simulink model "furuta_model"  (R2025a)
settings: Solver=VariableStepAuto  StartTime=0.0  StopTime=50  RelTol=1e-3
libraries: slpidlib x4
settings Model: Creator=deng_zhiwen  LastModifiedBy=deng_zhiwen

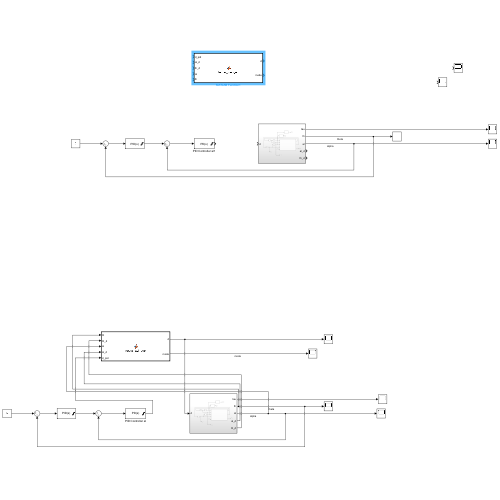
[thumbnail: Simulink's stored preview of the top-level diagram]
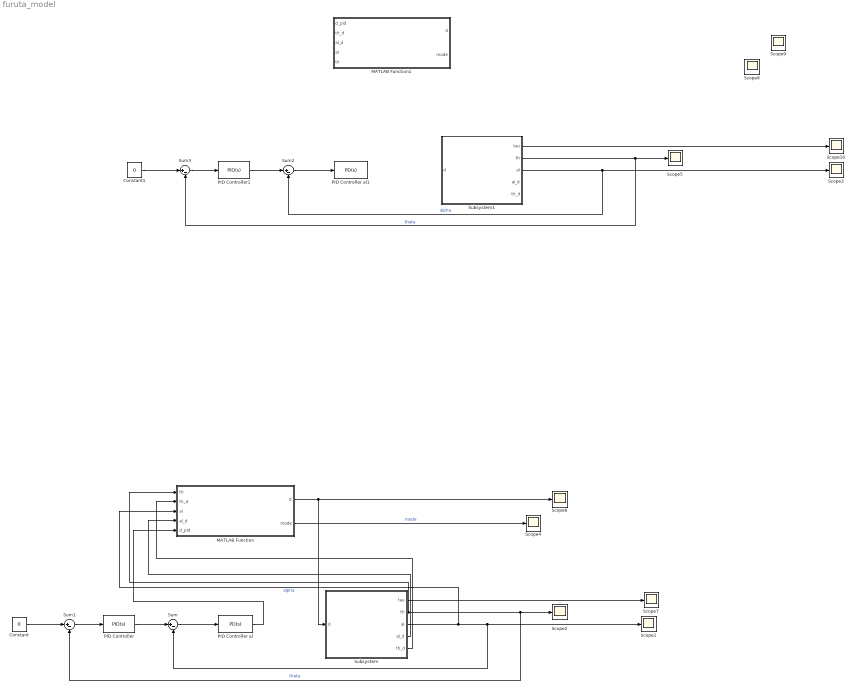
== system furuta_model ==
  Constant : Constant  Value=0
  Constant1 : Constant  Value=0
  MATLAB Function : MATLAB Function  TreatAsAtomicUnit=on
  MATLAB Function1 : MATLAB Function  TreatAsAtomicUnit=on
  PID Controller : slpidlib/PID Controller  Controller=PID  Form=Parallel  TimeDomain=Continuous-time  UseExternalTs=off  SampleTime=-1  IntegratorMethod=Forward Euler  FilterMethod=Forward Euler  ControllerParametersSource=internal  P=0.075  I=0.004  UseKiTs=off  D=0.041  UseExternalDerivativeSource=off  N=100  UseFilter=on  TunerSelectOption=Transfer Function Based (PID Tuner App)  InitialConditionSource=internal  InitialConditionForIntegrator=0  InitialConditionForFilter=0  DifferentiatorICPrevScaledInput=0  ExternalReset=none  TrackingMode=off  Kt=1  LimitOutput=on  SatLimitsSource=internal  UpperSaturationLimit=0.4  LowerSaturationLimit=-0.4  LinearizeAsGain=on  AntiWindupMode=none  Kb=1  LimitIntegrator=off  UpperIntegratorSaturationLimit=inf  LowerIntegratorSaturationLimit=-inf  POutMin=[]  POutMax=[]  IOutMin=[]  IOutMax=[]  DOutMin=[]  DOutMax=[]  NOutMin=[]  NOutMax=[]  SumOutMin=[]  SumOutMax=[]  SaturationOutMin=[]  SaturationOutMax=[]  PParamMin=[]  PParamMax=[]  IParamMin=[]  IParamMax=[]  DParamMin=[]  DParamMax=[]  NParamMin=[]  NParamMax=[]  KbParamMin=[]  KbParamMax=[]  KtParamMin=[]  KtParamMax=[]  KbOutMin=[]  KbOutMax=[]  KtOutMin=[]  KtOutMax=[]  IntegratorOutMin=[]  IntegratorOutMax=[]  FilterOutMin=[]  FilterOutMax=[]  SumI1OutMin=[]  SumI1OutMax=[]  SumI2OutMin=[]  SumI2OutMax=[]  SumI3OutMin=[]  SumI3OutMax=[]  SumI4OutMin=[]  SumI4OutMax=[]  SumDOutMin=[]  SumDOutMax=[]  DifferentiatorOutMin=[]  DifferentiatorOutMax=[]  FilterDiffOutCoefMin=[]  FilterDiffOutCoefMax=[]  ReciprocalOutMin=[]  ReciprocalOutMax=[]  SumDenOutMin=[]  SumDenOutMax=[]  SumNumOutMin=[]  SumNumOutMax=[]  DivideOutMin=[]  DivideOutMax=[]  UdiffTsProdOutMin=[]  UdiffTsProdOutMax=[]  NTsProdOutMin=[]  NTsProdOutMax=[]  UintegralTsProdOutMin=[]  UintegralTsProdOutMax=[]  UngainTsProdOutMin=[]  UngainTsProdOutMax=[]  ClampingZeroOutDataTypeStr=Inherit: Inherit via back propagation  ClampingZeroOutMin=[]  ClampingZeroOutMax=[]  FilterDenConstantOutDataTypeStr=Inherit: Inherit via back propagation  FilterDenConstantOutMin=[]  FilterDenConstantOutMax=[]  PCopyOutDataTypeStr=Inherit: Inherit via back propagation  PCopyOutMin=[]  PCopyOutMax=[]  NCopyOutDataTypeStr=Inherit: Inherit via back propagation  NCopyOutMin=[]  NCopyOutMax=[]  IntegratorContinuousStateAttributes=''  IntegratorStateMustResolveToSignalObject=off  IntegratorRTWStateStorageClass=Auto  FilterContinuousStateAttributes=''  FilterStateMustResolveToSignalObject=off  FilterRTWStateStorageClass=Auto  ParallelPVariant=InternalParameters  IdealPVariant=Disabled  IVariant=InternalParameters  DVariant=InternalParameters  IntegratorVariant=Continuous  SatVariant=Enabled  AWVariant=Passthrough  PCopyVariant=Disabled  TRVariant=Disabled  FdbkBlocksVariant=Forward  IdealPFdbkVariant=Disabled  SatFdbkVariant=Disabled  DerivativeFilterVariant=ContFilter  NVariant=InternalParameters  NCopyVariant=Disabled  FilterICVariant=InternalICsFilter  IntegratorICVariant=InternalICs  ExternalResetVariant=Disabled  TRSumVariant=Passthrough  SumFdbkVariant=Disabled  SumVariant=Sum_PID  TsampFilterVariant=InternalTs  TsampNgainVariant=Passthrough  TsampIntegralVariant=Disabled_SignalSpec  ExternalSaturationOutDataTypeStr=Inherit: Same as second input  DerivativeSourceVariant=ErrorSignal  PreIntVariant=InternalPreInt
  PID Controller al : slpidlib/PID Controller  Controller=PD  Form=Parallel  TimeDomain=Continuous-time  UseExternalTs=off  SampleTime=-1  IntegratorMethod=Forward Euler  FilterMethod=Forward Euler  ControllerParametersSource=internal  P=-1.37821105216692  I=-0.127510528430422  UseKiTs=off  D=-0.100817816501645  UseExternalDerivativeSource=off  N=47.2284869884382  UseFilter=on  TunerSelectOption=Transfer Function Based (PID Tuner App)  InitialConditionSource=internal  InitialConditionForIntegrator=0  InitialConditionForFilter=0  DifferentiatorICPrevScaledInput=0  ExternalReset=none  TrackingMode=off  Kt=1  LimitOutput=on  SatLimitsSource=internal  UpperSaturationLimit=1  LowerSaturationLimit=-1  LinearizeAsGain=on  AntiWindupMode=none  Kb=1  LimitIntegrator=off  UpperIntegratorSaturationLimit=inf  LowerIntegratorSaturationLimit=-inf  POutMin=[]  POutMax=[]  IOutMin=[]  IOutMax=[]  DOutMin=[]  DOutMax=[]  NOutMin=[]  NOutMax=[]  SumOutMin=[]  SumOutMax=[]  SaturationOutMin=[]  SaturationOutMax=[]  PParamMin=[]  PParamMax=[]  IParamMin=[]  IParamMax=[]  DParamMin=[]  DParamMax=[]  NParamMin=[]  NParamMax=[]  KbParamMin=[]  KbParamMax=[]  KtParamMin=[]  KtParamMax=[]  KbOutMin=[]  KbOutMax=[]  KtOutMin=[]  KtOutMax=[]  IntegratorOutMin=[]  IntegratorOutMax=[]  FilterOutMin=[]  FilterOutMax=[]  SumI1OutMin=[]  SumI1OutMax=[]  SumI2OutMin=[]  SumI2OutMax=[]  SumI3OutMin=[]  SumI3OutMax=[]  SumI4OutMin=[]  SumI4OutMax=[]  SumDOutMin=[]  SumDOutMax=[]  DifferentiatorOutMin=[]  DifferentiatorOutMax=[]  FilterDiffOutCoefMin=[]  FilterDiffOutCoefMax=[]  ReciprocalOutMin=[]  ReciprocalOutMax=[]  SumDenOutMin=[]  SumDenOutMax=[]  SumNumOutMin=[]  SumNumOutMax=[]  DivideOutMin=[]  DivideOutMax=[]  UdiffTsProdOutMin=[]  UdiffTsProdOutMax=[]  NTsProdOutMin=[]  NTsProdOutMax=[]  UintegralTsProdOutMin=[]  UintegralTsProdOutMax=[]  UngainTsProdOutMin=[]  UngainTsProdOutMax=[]  ClampingZeroOutDataTypeStr=Inherit: Inherit via back propagation  ClampingZeroOutMin=[]  ClampingZeroOutMax=[]  FilterDenConstantOutDataTypeStr=Inherit: Inherit via back propagation  FilterDenConstantOutMin=[]  FilterDenConstantOutMax=[]  PCopyOutDataTypeStr=Inherit: Inherit via back propagation  PCopyOutMin=[]  PCopyOutMax=[]  NCopyOutDataTypeStr=Inherit: Inherit via back propagation  NCopyOutMin=[]  NCopyOutMax=[]  IntegratorContinuousStateAttributes=''  IntegratorStateMustResolveToSignalObject=off  IntegratorRTWStateStorageClass=Auto  FilterContinuousStateAttributes=''  FilterStateMustResolveToSignalObject=off  FilterRTWStateStorageClass=Auto  ParallelPVariant=InternalParameters  IdealPVariant=Disabled  IVariant=Disabled  DVariant=InternalParameters  IntegratorVariant=Disabled  SatVariant=Enabled  AWVariant=Disabled  PCopyVariant=Disabled  TRVariant=Disabled  FdbkBlocksVariant=Forward  IdealPFdbkVariant=Disabled  SatFdbkVariant=Disabled  DerivativeFilterVariant=ContFilter  NVariant=InternalParameters  NCopyVariant=Disabled  FilterICVariant=InternalICsFilter  IntegratorICVariant=Disabled  ExternalResetVariant=Disabled  TRSumVariant=Passthrough  SumFdbkVariant=Disabled  SumVariant=Sum_PD  TsampFilterVariant=InternalTs  TsampNgainVariant=Passthrough  TsampIntegralVariant=Disabled_SignalSpec  ExternalSaturationOutDataTypeStr=Inherit: Same as second input  DerivativeSourceVariant=ErrorSignal  PreIntVariant=InternalPreInt
  PID Controller al1 : slpidlib/PID Controller  Controller=PD  Form=Parallel  TimeDomain=Continuous-time  UseExternalTs=off  SampleTime=-1  IntegratorMethod=Forward Euler  FilterMethod=Forward Euler  ControllerParametersSource=internal  P=-1.37821105216692  I=-0.127510528430422  UseKiTs=off  D=-0.100817816501645  UseExternalDerivativeSource=off  N=47.2284869884382  UseFilter=on  TunerSelectOption=Transfer Function Based (PID Tuner App)  InitialConditionSource=internal  InitialConditionForIntegrator=0  InitialConditionForFilter=0  DifferentiatorICPrevScaledInput=0  ExternalReset=none  TrackingMode=off  Kt=1  LimitOutput=on  SatLimitsSource=internal  UpperSaturationLimit=1  LowerSaturationLimit=-1  LinearizeAsGain=on  AntiWindupMode=none  Kb=1  LimitIntegrator=off  UpperIntegratorSaturationLimit=inf  LowerIntegratorSaturationLimit=-inf  POutMin=[]  POutMax=[]  IOutMin=[]  IOutMax=[]  DOutMin=[]  DOutMax=[]  NOutMin=[]  NOutMax=[]  SumOutMin=[]  SumOutMax=[]  SaturationOutMin=[]  SaturationOutMax=[]  PParamMin=[]  PParamMax=[]  IParamMin=[]  IParamMax=[]  DParamMin=[]  DParamMax=[]  NParamMin=[]  NParamMax=[]  KbParamMin=[]  KbParamMax=[]  KtParamMin=[]  KtParamMax=[]  KbOutMin=[]  KbOutMax=[]  KtOutMin=[]  KtOutMax=[]  IntegratorOutMin=[]  IntegratorOutMax=[]  FilterOutMin=[]  FilterOutMax=[]  SumI1OutMin=[]  SumI1OutMax=[]  SumI2OutMin=[]  SumI2OutMax=[]  SumI3OutMin=[]  SumI3OutMax=[]  SumI4OutMin=[]  SumI4OutMax=[]  SumDOutMin=[]  SumDOutMax=[]  DifferentiatorOutMin=[]  DifferentiatorOutMax=[]  FilterDiffOutCoefMin=[]  FilterDiffOutCoefMax=[]  ReciprocalOutMin=[]  ReciprocalOutMax=[]  SumDenOutMin=[]  SumDenOutMax=[]  SumNumOutMin=[]  SumNumOutMax=[]  DivideOutMin=[]  DivideOutMax=[]  UdiffTsProdOutMin=[]  UdiffTsProdOutMax=[]  NTsProdOutMin=[]  NTsProdOutMax=[]  UintegralTsProdOutMin=[]  UintegralTsProdOutMax=[]  UngainTsProdOutMin=[]  UngainTsProdOutMax=[]  ClampingZeroOutDataTypeStr=Inherit: Inherit via back propagation  ClampingZeroOutMin=[]  ClampingZeroOutMax=[]  FilterDenConstantOutDataTypeStr=Inherit: Inherit via back propagation  FilterDenConstantOutMin=[]  FilterDenConstantOutMax=[]  PCopyOutDataTypeStr=Inherit: Inherit via back propagation  PCopyOutMin=[]  PCopyOutMax=[]  NCopyOutDataTypeStr=Inherit: Inherit via back propagation  NCopyOutMin=[]  NCopyOutMax=[]  IntegratorContinuousStateAttributes=''  IntegratorStateMustResolveToSignalObject=off  IntegratorRTWStateStorageClass=Auto  FilterContinuousStateAttributes=''  FilterStateMustResolveToSignalObject=off  FilterRTWStateStorageClass=Auto  ParallelPVariant=InternalParameters  IdealPVariant=Disabled  IVariant=Disabled  DVariant=InternalParameters  IntegratorVariant=Disabled  SatVariant=Enabled  AWVariant=Disabled  PCopyVariant=Disabled  TRVariant=Disabled  FdbkBlocksVariant=Forward  IdealPFdbkVariant=Disabled  SatFdbkVariant=Disabled  DerivativeFilterVariant=ContFilter  NVariant=InternalParameters  NCopyVariant=Disabled  FilterICVariant=InternalICsFilter  IntegratorICVariant=Disabled  ExternalResetVariant=Disabled  TRSumVariant=Passthrough  SumFdbkVariant=Disabled  SumVariant=Sum_PD  TsampFilterVariant=InternalTs  TsampNgainVariant=Passthrough  TsampIntegralVariant=Disabled_SignalSpec  ExternalSaturationOutDataTypeStr=Inherit: Same as second input  DerivativeSourceVariant=ErrorSignal  PreIntVariant=InternalPreInt
  PID Controller1 : slpidlib/PID Controller  Controller=PID  Form=Parallel  TimeDomain=Continuous-time  UseExternalTs=off  SampleTime=-1  IntegratorMethod=Forward Euler  FilterMethod=Forward Euler  ControllerParametersSource=internal  P=0.075  I=0.004  UseKiTs=off  D=0.041  UseExternalDerivativeSource=off  N=100  UseFilter=on  TunerSelectOption=Transfer Function Based (PID Tuner App)  InitialConditionSource=internal  InitialConditionForIntegrator=0  InitialConditionForFilter=0  DifferentiatorICPrevScaledInput=0  ExternalReset=none  TrackingMode=off  Kt=1  LimitOutput=on  SatLimitsSource=internal  UpperSaturationLimit=0.4  LowerSaturationLimit=-0.4  LinearizeAsGain=on  AntiWindupMode=none  Kb=1  LimitIntegrator=off  UpperIntegratorSaturationLimit=inf  LowerIntegratorSaturationLimit=-inf  POutMin=[]  POutMax=[]  IOutMin=[]  IOutMax=[]  DOutMin=[]  DOutMax=[]  NOutMin=[]  NOutMax=[]  SumOutMin=[]  SumOutMax=[]  SaturationOutMin=[]  SaturationOutMax=[]  PParamMin=[]  PParamMax=[]  IParamMin=[]  IParamMax=[]  DParamMin=[]  DParamMax=[]  NParamMin=[]  NParamMax=[]  KbParamMin=[]  KbParamMax=[]  KtParamMin=[]  KtParamMax=[]  KbOutMin=[]  KbOutMax=[]  KtOutMin=[]  KtOutMax=[]  IntegratorOutMin=[]  IntegratorOutMax=[]  FilterOutMin=[]  FilterOutMax=[]  SumI1OutMin=[]  SumI1OutMax=[]  SumI2OutMin=[]  SumI2OutMax=[]  SumI3OutMin=[]  SumI3OutMax=[]  SumI4OutMin=[]  SumI4OutMax=[]  SumDOutMin=[]  SumDOutMax=[]  DifferentiatorOutMin=[]  DifferentiatorOutMax=[]  FilterDiffOutCoefMin=[]  FilterDiffOutCoefMax=[]  ReciprocalOutMin=[]  ReciprocalOutMax=[]  SumDenOutMin=[]  SumDenOutMax=[]  SumNumOutMin=[]  SumNumOutMax=[]  DivideOutMin=[]  DivideOutMax=[]  UdiffTsProdOutMin=[]  UdiffTsProdOutMax=[]  NTsProdOutMin=[]  NTsProdOutMax=[]  UintegralTsProdOutMin=[]  UintegralTsProdOutMax=[]  UngainTsProdOutMin=[]  UngainTsProdOutMax=[]  ClampingZeroOutDataTypeStr=Inherit: Inherit via back propagation  ClampingZeroOutMin=[]  ClampingZeroOutMax=[]  FilterDenConstantOutDataTypeStr=Inherit: Inherit via back propagation  FilterDenConstantOutMin=[]  FilterDenConstantOutMax=[]  PCopyOutDataTypeStr=Inherit: Inherit via back propagation  PCopyOutMin=[]  PCopyOutMax=[]  NCopyOutDataTypeStr=Inherit: Inherit via back propagation  NCopyOutMin=[]  NCopyOutMax=[]  IntegratorContinuousStateAttributes=''  IntegratorStateMustResolveToSignalObject=off  IntegratorRTWStateStorageClass=Auto  FilterContinuousStateAttributes=''  FilterStateMustResolveToSignalObject=off  FilterRTWStateStorageClass=Auto  ParallelPVariant=InternalParameters  IdealPVariant=Disabled  IVariant=InternalParameters  DVariant=InternalParameters  IntegratorVariant=Continuous  SatVariant=Enabled  AWVariant=Passthrough  PCopyVariant=Disabled  TRVariant=Disabled  FdbkBlocksVariant=Forward  IdealPFdbkVariant=Disabled  SatFdbkVariant=Disabled  DerivativeFilterVariant=ContFilter  NVariant=InternalParameters  NCopyVariant=Disabled  FilterICVariant=InternalICsFilter  IntegratorICVariant=InternalICs  ExternalResetVariant=Disabled  TRSumVariant=Passthrough  SumFdbkVariant=Disabled  SumVariant=Sum_PID  TsampFilterVariant=InternalTs  TsampNgainVariant=Passthrough  TsampIntegralVariant=Disabled_SignalSpec  ExternalSaturationOutDataTypeStr=Inherit: Same as second input  DerivativeSourceVariant=ErrorSignal  PreIntVariant=InternalPreInt
  Scope{1..10} (10 alike) : Scope
      Scope1 settings: ActiveDisplayYMinimum=-3.9269908169872414  ActiveDisplayYMaximum=3.9269908169872414
      Scope10 settings: ActiveDisplayYMinimum=-1  ActiveDisplayYMaximum=1  DataLoggingVariableName=ScopeData3
      Scope2 settings: ActiveDisplayYMinimum=-3.9269908169872245  ActiveDisplayYMaximum=3.926990816987229  DataLoggingVariableName=ScopeData2
      Scope3 settings: ActiveDisplayYMinimum=-3.9269908169872414  ActiveDisplayYMaximum=3.9269908169872414  DataLoggingVariableName=ScopeData4
      Scope4 settings: ActiveDisplayYMinimum=-0.15834947271429556  ActiveDisplayYMaximum=1.034336584628718
      Scope5 settings: ActiveDisplayYMinimum=-3.9269908169872245  ActiveDisplayYMaximum=3.926990816987229  DataLoggingVariableName=ScopeData5
      Scope6 settings: ActiveDisplayYMinimum=-1.4910481407596079  ActiveDisplayYMaximum=1.3792930645972798  DataLoggingVariableName=ScopeData6
      Scope7 settings: ActiveDisplayYMinimum=-1  ActiveDisplayYMaximum=1  DataLoggingVariableName=ScopeData7
      Scope8 settings: ActiveDisplayYMinimum=-0.15834947271429556  ActiveDisplayYMaximum=1.034336584628718  DataLoggingVariableName=ScopeData8
      Scope9 settings: ActiveDisplayYMinimum=-1.4910481407596079  ActiveDisplayYMaximum=1.3792930645972798  DataLoggingVariableName=ScopeData9
  Subsystem : Subsystem
  Subsystem1 : Subsystem
  Sum{,1..3} (4 alike) : Sum  Inputs=|+-
  wires:
  Subsystem/2(th) -> MATLAB Function/1(th), Sum1/2, Scope2/1  "theta"
  Constant/1 -> Sum1/1
  PID Controller/1 -> Sum/1
  Sum1/1 -> PID Controller/1
  Sum/1 -> PID Controller al/1
  Subsystem/3(al) -> Sum/2, Scope1/1, MATLAB Function/3(al)  "alpha"
  Subsystem/5(th_d) -> MATLAB Function/2(th_d)
  Subsystem/4(al_d) -> MATLAB Function/4(al_d)
  MATLAB Function/1(d) -> Scope6/1, Subsystem/1(d)
  PID Controller al/1 -> MATLAB Function/5(d_pid)
  MATLAB Function/2(mode) -> Scope4/1  "mode"
  Subsystem/1(tau) -> Scope7/1
  Subsystem1/2(th) -> Sum3/2, Scope5/1  "theta"
  PID Controller1/1 -> Sum2/1
  Subsystem1/1(tau) -> Scope10/1
  Constant1/1 -> Sum3/1
  Sum3/1 -> PID Controller1/1
  Subsystem1/3(al) -> Sum2/2, Scope3/1  "alpha"
  Sum2/1 -> PID Controller al1/1

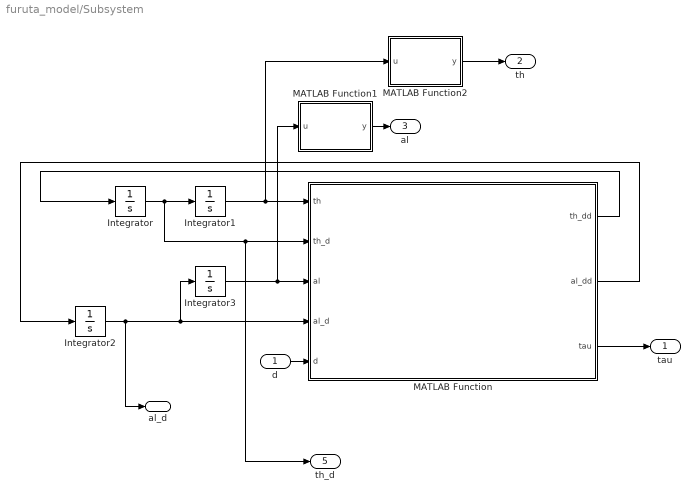
== system furuta_model/Subsystem ==
  d : Inport
  Integrator : Integrator
  Integrator1 : Integrator
  Integrator2 : Integrator  InitialCondition=0.3
  Integrator3 : Integrator  InitialCondition=0.24
  MATLAB Function : MATLAB Function  TreatAsAtomicUnit=on
  MATLAB Function1 : MATLAB Function  TreatAsAtomicUnit=on
  MATLAB Function2 : MATLAB Function  TreatAsAtomicUnit=on
  tau : Outport
  th : Outport  Port=2
  al : Outport  Port=3
  al_d : Outport  Port=4
  th_d : Outport  Port=5
  wires:
  MATLAB Function/1(th_dd) -> Integrator/1
  MATLAB Function/2(al_dd) -> Integrator2/1
  Integrator/1 -> Integrator1/1, MATLAB Function/2(th_d), th_d/1
  d/1 -> MATLAB Function/5(d)
  Integrator2/1 -> MATLAB Function/4(al_d), Integrator3/1, al_d/1
  MATLAB Function/3(tau) -> tau/1
  Integrator1/1 -> MATLAB Function2/1(u), MATLAB Function/1(th)
  Integrator3/1 -> MATLAB Function1/1(u), MATLAB Function/3(al)
  MATLAB Function1/1(y) -> al/1
  MATLAB Function2/1(y) -> th/1

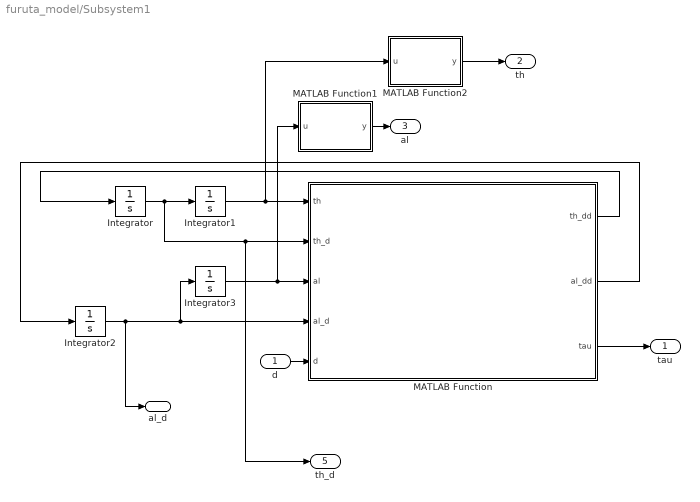
== system furuta_model/Subsystem1 ==
  d : Inport
  Integrator : Integrator
  Integrator1 : Integrator
  Integrator2 : Integrator  InitialCondition=0.3
  Integrator3 : Integrator  InitialCondition=0.24
  MATLAB Function : MATLAB Function  TreatAsAtomicUnit=on
  MATLAB Function1 : MATLAB Function  TreatAsAtomicUnit=on
  MATLAB Function2 : MATLAB Function  TreatAsAtomicUnit=on
  tau : Outport
  th : Outport  Port=2
  al : Outport  Port=3
  al_d : Outport  Port=4
  th_d : Outport  Port=5
  wires:
  MATLAB Function/1(th_dd) -> Integrator/1
  MATLAB Function/2(al_dd) -> Integrator2/1
  Integrator/1 -> Integrator1/1, MATLAB Function/2(th_d), th_d/1
  d/1 -> MATLAB Function/5(d)
  Integrator2/1 -> MATLAB Function/4(al_d), Integrator3/1, al_d/1
  MATLAB Function/3(tau) -> tau/1
  Integrator1/1 -> MATLAB Function2/1(u), MATLAB Function/1(th)
  Integrator3/1 -> MATLAB Function1/1(u), MATLAB Function/3(al)
  MATLAB Function1/1(y) -> al/1
  MATLAB Function2/1(y) -> th/1

== matlab function furuta_model/Subsystem/MATLAB Function1 ==
  data: u input; y output
function y = wrap_angle(u)
    y = atan2(sin(u), cos(u));
end

== matlab function furuta_model/Subsystem/MATLAB Function ==
  data: th input; th_dd output; th_d input; al input; al_d input; d input; al_dd output; tau output
function [th_dd, al_dd, tau] = furuta_step(th, th_d, al, al_d, d)
%#codegen
% States: th=theta, th_d=theta_dot, al=alpha, al_d=alpha_dot
% Input:  d = PWM duty [-1, 1]
% Output: th_dd, al_dd [rad/s²], tau [N·m]

% -------------------------------------------------------------------------
% 物理参数
% -------------------------------------------------------------------------
J_theta = 2.5e-4;   % 旋转臂转动惯量        [kg·m²]
J_alpha = 1.2e-3;   % 摆杆转动惯量          [kg·m²]
m_p     = 0.120;    % 摆杆质量              [kg]
r       = 0.1;      % 旋转臂长度            [m]
l       = 0.1;      % 摆杆质心到摆轴距离    [m]
g       = 9.81;     % 重力加速度            [m/s²]
B_r     = 0.0024;   % 旋转臂阻尼系数        [N·m·s/rad]
B_p     = 0.0024;   % 摆轴阻尼系数          [N·m·s/rad]

% 电机参数
K_g     = 9.2767;   % 减速比
V_s     = 5.0;      % 供电电压              [V]
R_m     = 2.5;      % 电枢电阻              [Ω]
k_t     = 0.020;    % 力矩常数              [N·m/A]
k_e     = 0.020;    % 反电动势常数          [V·s/rad]
eta_m   = 0.7;      % 电机效率
eta_g   = 0.7;      % 减速箱效率
tau_max = 0.25;     % 力矩饱和值            [N·m]

% -------------------------------------------------------------------------
% 动力学方程组合参数（从物理参数推导，便于核查）
%
%   惯性矩阵 M = [a,        e*cos(al)]
%               [e*cos(al), c        ]
%
%   a  = J_theta + m_p*r²   旋转臂等效惯量
%   c  = J_alpha + m_p*l²   摆杆等效惯量
%   e  = m_p*r*l            耦合项幅值，实际耦合项 b = e*cos(al)
%   g0 = m_p*g*l            重力项幅值，实际重力项 = g0*sin(al)
% -------------------------------------------------------------------------
a  = J_theta + m_p * r^2;   % = 2.5e-4 + 0.12×0.1² = 1.45e-3  [kg·m²]
c  = J_alpha + m_p * l^2;   % = 1.2e-3 + 0.12×0.1² = 2.40e-3  [kg·m²]
e  = m_p * r * l;           % = 0.12×0.1×0.1        = 1.20e-3  [kg·m²]
g0 = m_p * g * l;           % = 0.12×9.81×0.1       = 0.11772  [N·m]

% -------------------------------------------------------------------------
% 力矩计算: tau = eta_m*eta_g*K_g*k_t*(V_s*d - k_e*K_g*th_d) / R_m
%               = Cd*d - Cv*th_d
% -------------------------------------------------------------------------
Cd = eta_m * eta_g * K_g * k_t * V_s / R_m;       % ≈ 0.18182 [N·m/duty]
Cv = eta_m * eta_g * K_g^2 * k_t * k_e / R_m;     % ≈ 0.00675 [N·m·s/rad]

tau_raw = Cd*d - Cv*th_d;
tau     = max(-tau_max, min(tau_max, tau_raw));     % 力矩饱和
% -------------------------------------------------------------------------
% 构建右端向量
%
%   rhs1 = tau - B_r*th_d + e*sin(al)*al_d²    (θ方程，含离心项)
%   rhs2 =     - B_p*al_d + g0*sin(al)          (α方程，含重力项)
% -------------------------------------------------------------------------
b    = e * cos(al);                        % 惯性矩阵耦合项    [kg·m²]

rhs1 = tau - B_r*th_d + e*sin(al)*al_d^2;
rhs2 =     - B_p*al_d + g0*sin(al);

% -------------------------------------------------------------------------
% 克莱姆法则求解 M*[th_dd; al_dd] = [rhs1; rhs2]
%
%   detM = a*c - b²  (恒 > 0，已验证最小值 a*c-e² = 2.04e-6 > 0)
% -------------------------------------------------------------------------
detM  = a*c - b^2;

th_dd = ( c*rhs1 - b*rhs2) / detM;
al_dd = (-b*rhs1 + a*rhs2) / detM;

end

== matlab function furuta_model/Subsystem/MATLAB Function2 ==
  data: u input; y output
function y = wrap_angle(u)
    y = atan2(sin(u), cos(u));
end

== matlab function furuta_model/MATLAB Function ==
  data: th input; d output; th_d input; al input; al_d input; d_pid input; mode output
function [d, mode] = furuta_swingup(th, th_d, al, al_d, d_pid)
%#codegen
% Inputs:
%   th, th_d : 旋转臂角度和角速度 [rad, rad/s]
%   al, al_d : 摆杆角度和角速度 [rad, rad/s] (al=0为倒立，al=+-pi为自然下垂)
%   d_pid    : PID控制器计算出的占空比 (用于在起摆完成后接管)
% Outputs:
%   d        : 最终输出给电机的占空比 [-1, 1]
%   mode     : 当前控制模式 (0: 起摆模式, 1: PID稳态控制模式)

% --- 关键修复：显式初始化输出变量的维度和类型，防止Simulink报错 ---
d = 0.0;
mode = 0;

% -------------------------------------------------------------------------
% 物理参数 (与你的动力学模型完全一致)
% -------------------------------------------------------------------------
J_theta = 2.5e-4;   
J_alpha = 1.2e-3;   
m_p     = 0.120;    
r       = 0.1;      
l       = 0.1;      
g       = 9.81;     
B_r     = 0.0024;   
B_p     = 0.0024;   

% 电机参数
K_g     = 9.2767;   
V_s     = 5.0;      
R_m     = 2.5;      
k_t     = 0.020;    
k_e     = 0.020;    
eta_m   = 0.7;      
eta_g   = 0.7;      

% 动力学组合参数
a  = J_theta + m_p * r^2;
c  = J_alpha + m_p * l^2;
e  = m_p * r * l;
g0 = m_p * g * l;

% 电机模型组合参数
Cd = eta_m * eta_g * K_g * k_t * V_s / R_m;
Cv = eta_m * eta_g * K_g^2 * k_t * k_e / R_m;

% -------------------------------------------------------------------------
% 1. 角度规范化到 [-pi, pi]
% -------------------------------------------------------------------------
% 防止由于多圈旋转导致的角度累加，将 al 限制在 [-pi, pi]
al_wrap = mod(al + pi, 2*pi) - pi;

% -------------------------------------------------------------------------
% 2. 切换逻辑：判断是否进入PID接管范围 (20度)
% -------------------------------------------------------------------------
threshold = 20 * pi / 180; % 20度转化为弧度

if abs(al_wrap) <= threshold
    % --- PID 接管模式 ---
    mode = 1; 
    d = d_pid;
else
    % --- 能量起摆模式 ---
    mode = 0; 
    
    % ---------------------------------------------------------------------
    % 3. 满血版 Bang-Bang 能量控制律 (解决高处回落问题)
    % ---------------------------------------------------------------------
    E = 0.5 * c * al_d^2 + g0 * cos(al);
    
    % 【关键修改1】将目标能量提高到理论最大势能的 1.5 倍！
    % 防止在接近最高点时，控制器认为“能量够了”而提前关断电机，导致被摩擦力消耗掉而掉下来。
    E0 = g0 * 1.5; 
    
    k_acc = 120.0; 
    
    % 【关键修改2】限制旋臂回中力矩的最大值
    % 防止旋臂偏离过大时，PD控制力矩增长过大，喧宾夺主抵消了起摆力矩
    pd_term = 2.0 * th + 2.0 * th_d;
    pd_term = max(-50, min(50, pd_term)); % 强行限幅
    
    pump_direction = sign(al_d * cos(al));
    if pump_direction == 0
        pump_direction = 1; 
    end
    
    % 只要能量不够，就全功率泵入 (由于 E0 设得很高，起摆阶段会一直全功率泵入)
    if E < E0
        th_dd_cmd = -k_acc * pump_direction - pd_term;
    else
        th_dd_cmd = -pd_term; 
    end
    
    % 限制期望加速度
    th_dd_cmd = max(-150, min(150, th_dd_cmd));

    
    % ---------------------------------------------------------------------
    % 4. 逆动力学补偿计算目标力矩 (tau_cmd)
    % ---------------------------------------------------------------------
    b = e * cos(al);
    
    % 根据期望的 th_dd_cmd 预测此时摆杆的角加速度 al_dd
    % 由动力学方程2变形得到: c * al_dd = -b * th_dd - B_p * al_d + g0 * sin(al)
    al_dd_pred = (-b * th_dd_cmd - B_p * al_d + g0 * sin(al)) / c;
    
    % 代入动力学方程1求所需的目标力矩 tau_cmd
    % a * th_dd + b * al_dd = tau - B_r * th_d + e * sin(al) * al_d^2
    tau_cmd = a * th_dd_cmd + b * al_dd_pred + B_r * th_d - e * sin(al) * al_d^2;
    
    % ---------------------------------------------------------------------
    % 5. 逆电机模型补偿计算占空比 (d)
    % ---------------------------------------------------------------------
    % 正向电机模型: tau = Cd * d - Cv * th_d
    % 逆向电机模型: d = (tau + Cv * th_d) / Cd
    d_raw = (tau_cmd + Cv * th_d) / Cd;
    
    % 占空比饱和限制 [-1, 1]
    d = max(-1, min(1, d_raw));
end

end

== matlab function furuta_model/MATLAB Function1 ==
  data: d_pid input; th_d input; al_d input; al input; th input; d output; mode output
function [d, mode] = furuta_swingup(d_pid,th_d,al_d,al,th)
%#codegen
% Inputs:
%   th, th_d : 旋转臂角度和角速度 [rad, rad/s]
%   al, al_d : 摆杆角度和角速度 [rad, rad/s] (al=0为倒立，al=+-pi为自然下垂)
%   d_pid    : PID控制器计算出的占空比 (用于在起摆完成后接管)
% Outputs:
%   d        : 最终输出给电机的占空比 [-1, 1]
%   mode     : 当前控制模式 (0: 起摆模式, 1: PID稳态控制模式)

% --- 关键修复：显式初始化输出变量的维度和类型，防止Simulink报错 ---
d = 0.0;
mode = 0;

% -------------------------------------------------------------------------
% 物理参数 (与你的动力学模型完全一致)
% -------------------------------------------------------------------------
J_theta = 2.5e-4;   
J_alpha = 1.2e-3;   
m_p     = 0.120;    
r       = 0.1;      
l       = 0.1;      
g       = 9.81;     
B_r     = 0.0024;   
B_p     = 0.0024;   

% 电机参数
K_g     = 9.2767;   
V_s     = 5.0;      
R_m     = 2.5;      
k_t     = 0.020;    
k_e     = 0.020;    
eta_m   = 0.7;      
eta_g   = 0.7;      

% 动力学组合参数
a  = J_theta + m_p * r^2;
c  = J_alpha + m_p * l^2;
e  = m_p * r * l;
g0 = m_p * g * l;

% 电机模型组合参数
Cd = eta_m * eta_g * K_g * k_t * V_s / R_m;
Cv = eta_m * eta_g * K_g^2 * k_t * k_e / R_m;

% -------------------------------------------------------------------------
% 1. 角度规范化到 [-pi, pi]
% -------------------------------------------------------------------------
% 防止由于多圈旋转导致的角度累加，将 al 限制在 [-pi, pi]
al_wrap = mod(al + pi, 2*pi) - pi;

% -------------------------------------------------------------------------
% 2. 切换逻辑：判断是否进入PID接管范围 (20度)
% -------------------------------------------------------------------------
threshold = 20 * pi / 180; % 20度转化为弧度

if abs(al_wrap) <= threshold
    % --- PID 接管模式 ---
    mode = 1; 
    d = d_pid;
else
    % --- 能量起摆模式 ---
    mode = 0; 
    
    % ---------------------------------------------------------------------
    % 3. 满血版 Bang-Bang 能量控制律 (解决高处回落问题)
    % ---------------------------------------------------------------------
    E = 0.5 * c * al_d^2 + g0 * cos(al);
    
    % 【关键修改1】将目标能量提高到理论最大势能的 1.5 倍！
    % 防止在接近最高点时，控制器认为“能量够了”而提前关断电机，导致被摩擦力消耗掉而掉下来。
    E0 = g0 * 1.5; 
    
    k_acc = 120.0; 
    
    % 【关键修改2】限制旋臂回中力矩的最大值
    % 防止旋臂偏离过大时，PD控制力矩增长过大，喧宾夺主抵消了起摆力矩
    pd_term = 2.0 * th + 2.0 * th_d;
    pd_term = max(-50, min(50, pd_term)); % 强行限幅
    
    pump_direction = sign(al_d * cos(al));
    if pump_direction == 0
        pump_direction = 1; 
    end
    
    % 只要能量不够，就全功率泵入 (由于 E0 设得很高，起摆阶段会一直全功率泵入)
    if E < E0
        th_dd_cmd = -k_acc * pump_direction - pd_term;
    else
        th_dd_cmd = -pd_term; 
    end
    
    % 限制期望加速度
    th_dd_cmd = max(-150, min(150, th_dd_cmd));

    
    % ---------------------------------------------------------------------
    % 4. 逆动力学补偿计算目标力矩 (tau_cmd)
    % ---------------------------------------------------------------------
    b = e * cos(al);
    
    % 根据期望的 th_dd_cmd 预测此时摆杆的角加速度 al_dd
    % 由动力学方程2变形得到: c * al_dd = -b * th_dd - B_p * al_d + g0 * sin(al)
    al_dd_pred = (-b * th_dd_cmd - B_p * al_d + g0 * sin(al)) / c;
    
    % 代入动力学方程1求所需的目标力矩 tau_cmd
    % a * th_dd + b * al_dd = tau - B_r * th_d + e * sin(al) * al_d^2
    tau_cmd = a * th_dd_cmd + b * al_dd_pred + B_r * th_d - e * sin(al) * al_d^2;
    
    % ---------------------------------------------------------------------
    % 5. 逆电机模型补偿计算占空比 (d)
    % ---------------------------------------------------------------------
    % 正向电机模型: tau = Cd * d - Cv * th_d
    % 逆向电机模型: d = (tau + Cv * th_d) / Cd
    d_raw = (tau_cmd + Cv * th_d) / Cd;
    
    % 占空比饱和限制 [-1, 1]
    d = max(-1, min(1, d_raw));
end

end

== matlab function furuta_model/Subsystem1/MATLAB Function ==
  data: th input; th_dd output; th_d input; al input; al_d input; d input; al_dd output; tau output
function [th_dd, al_dd, tau] = furuta_step(th, th_d, al, al_d, d)
%#codegen
% States: th=theta, th_d=theta_dot, al=alpha, al_d=alpha_dot
% Input:  d = PWM duty [-1, 1]
% Output: th_dd, al_dd [rad/s²], tau [N·m]

% -------------------------------------------------------------------------
% 物理参数
% -------------------------------------------------------------------------
J_theta = 2.5e-4;   % 旋转臂转动惯量        [kg·m²]
J_alpha = 1.2e-3;   % 摆杆转动惯量          [kg·m²]
m_p     = 0.120;    % 摆杆质量              [kg]
r       = 0.1;      % 旋转臂长度            [m]
l       = 0.1;      % 摆杆质心到摆轴距离    [m]
g       = 9.81;     % 重力加速度            [m/s²]
B_r     = 0.0024;   % 旋转臂阻尼系数        [N·m·s/rad]
B_p     = 0.0024;   % 摆轴阻尼系数          [N·m·s/rad]

% 电机参数
K_g     = 9.2767;   % 减速比
V_s     = 5.0;      % 供电电压              [V]
R_m     = 2.5;      % 电枢电阻              [Ω]
k_t     = 0.020;    % 力矩常数              [N·m/A]
k_e     = 0.020;    % 反电动势常数          [V·s/rad]
eta_m   = 0.7;      % 电机效率
eta_g   = 0.7;      % 减速箱效率
tau_max = 0.25;     % 力矩饱和值            [N·m]

% -------------------------------------------------------------------------
% 动力学方程组合参数（从物理参数推导，便于核查）
%
%   惯性矩阵 M = [a,        e*cos(al)]
%               [e*cos(al), c        ]
%
%   a  = J_theta + m_p*r²   旋转臂等效惯量
%   c  = J_alpha + m_p*l²   摆杆等效惯量
%   e  = m_p*r*l            耦合项幅值，实际耦合项 b = e*cos(al)
%   g0 = m_p*g*l            重力项幅值，实际重力项 = g0*sin(al)
% -------------------------------------------------------------------------
a  = J_theta + m_p * r^2;   % = 2.5e-4 + 0.12×0.1² = 1.45e-3  [kg·m²]
c  = J_alpha + m_p * l^2;   % = 1.2e-3 + 0.12×0.1² = 2.40e-3  [kg·m²]
e  = m_p * r * l;           % = 0.12×0.1×0.1        = 1.20e-3  [kg·m²]
g0 = m_p * g * l;           % = 0.12×9.81×0.1       = 0.11772  [N·m]

% -------------------------------------------------------------------------
% 力矩计算: tau = eta_m*eta_g*K_g*k_t*(V_s*d - k_e*K_g*th_d) / R_m
%               = Cd*d - Cv*th_d
% -------------------------------------------------------------------------
Cd = eta_m * eta_g * K_g * k_t * V_s / R_m;       % ≈ 0.18182 [N·m/duty]
Cv = eta_m * eta_g * K_g^2 * k_t * k_e / R_m;     % ≈ 0.00675 [N·m·s/rad]

tau_raw = Cd*d - Cv*th_d;
tau     = max(-tau_max, min(tau_max, tau_raw));     % 力矩饱和
% -------------------------------------------------------------------------
% 构建右端向量
%
%   rhs1 = tau - B_r*th_d + e*sin(al)*al_d²    (θ方程，含离心项)
%   rhs2 =     - B_p*al_d + g0*sin(al)          (α方程，含重力项)
% -------------------------------------------------------------------------
b    = e * cos(al);                        % 惯性矩阵耦合项    [kg·m²]

rhs1 = tau - B_r*th_d + e*sin(al)*al_d^2;
rhs2 =     - B_p*al_d + g0*sin(al);

% -------------------------------------------------------------------------
% 克莱姆法则求解 M*[th_dd; al_dd] = [rhs1; rhs2]
%
%   detM = a*c - b²  (恒 > 0，已验证最小值 a*c-e² = 2.04e-6 > 0)
% -------------------------------------------------------------------------
detM  = a*c - b^2;

th_dd = ( c*rhs1 - b*rhs2) / detM;
al_dd = (-b*rhs1 + a*rhs2) / detM;

end

== matlab function furuta_model/Subsystem1/MATLAB Function1 ==
  data: u input; y output
function y = wrap_angle(u)
    y = atan2(sin(u), cos(u));
end

== matlab function furuta_model/Subsystem1/MATLAB Function2 ==
  data: u input; y output
function y = wrap_angle(u)
    y = atan2(sin(u), cos(u));
end
